simulink model "class20"  (R2025b)
settings: Solver=VariableStepAuto  StartTime=0.0  StopTime=2  RelTol=1e-3
values from neighbouring files (symbols this model uses):
  K = lqr(A,B,Q,R)    [class10.m]    (also in class11.m; class21.m; class5.m = [0 0 1]*inv(cm)*phi_A; class8.m = place(A,B,p))
settings Model: Creator=anish  LastModifiedBy=anish

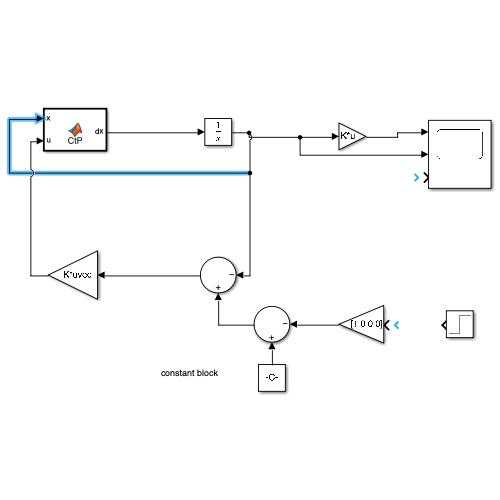
[thumbnail: Simulink's stored preview of the top-level diagram]
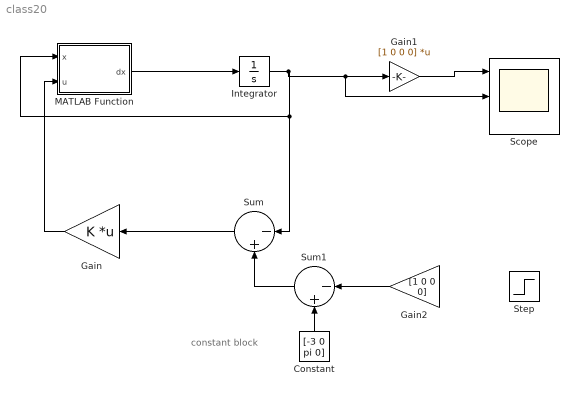
== system class20 ==
  note: constant block
  Constant : Constant  Value=[-3 0 pi 0]
  Gain : Gain  Gain=K  Multiplication=Matrix(K*u) (u vector)
  Gain1 : Gain  Gain=[1 0 0 0]  Multiplication=Matrix(K*u)
  Gain2 : Gain  Gain=[1 0 0 0]
  Integrator : Integrator  InitialCondition=[-4;0; pi; 0]
  MATLAB Function : MATLAB Function  TreatAsAtomicUnit=on
  Scope : Scope  NumInputPorts=3
      settings: ActiveDisplayYMinimum=-43.166175068843089  ActiveDisplayYMaximum=17.646490750945095
  Step : Step  SampleTime=1
  Sum : Sum  Inputs=|-+
  Sum1 : Sum  Inputs=|-+
  wires:
  MATLAB Function/1(dx) -> Integrator/1
  Gain/1 -> MATLAB Function/2(u)
  Integrator/1 -> Scope/2, Gain1/1, MATLAB Function/1(x), Sum/1
  Sum/1 -> Gain/1
  Gain1/1 -> Scope/1
  Constant/1 -> Sum1/2
  Gain2/1 -> Sum1/1
  Sum1/1 -> Sum/2

== matlab function class20/MATLAB Function ==
  data: x input; u input; dx output
function dx = CtP (x,u)

  dx = zeros(4,1);
  m = 1;
  M = 5; 
  L = 2; % length of pendulum
  g = -9.81; % m/s^2
  d = 1; % Ns/m

  Sx= sin(x(3));
  Cx = cos(x(3));
  D = m*L*L*(M+m*(1-Cx^2));

  dx(1,1) = x(2);
  dx(2,1) = (1/D)*(-m^2*L^2*g*Cx*Sx + m*L^2*(m*L*x(4)^2*Sx-d*x(2)))+m*L^2/D*u;
  dx(3,1) = x(4);
  dx(4,1) = (1/D)*((m+M)*m*g*L*Sx - m*L*Cx*(m*L*x(4)^2*Sx-d*x(2))) - m*L*Cx/D*u;

end
